simulink model "prey_pred_ext"  (R2023b)
settings: Solver=VariableStepAuto  StartTime=0.0  StopTime=tFinal  RelTol=1e-3
values from neighbouring files (symbols this model uses):
  a1 = 1    [prey_pred_ext_params.m]
  a2 = 1    [prey_pred_ext_params.m]
  b1 = 0.0002    [prey_pred_ext_params.m]
  g1 = 0.01    [prey_pred_ext_params.m]
  g2 = 0.001    [prey_pred_ext_params.m]
  x10 = 3000    [prey_pred_ext_params.m]
  x20 = 1000    [prey_pred_ext_params.m]
settings Model: Creator=martinhaugen  LastModifiedBy=martinhaugen

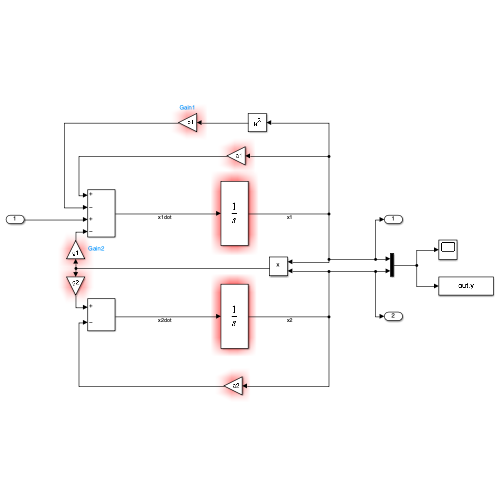
[thumbnail: Simulink's stored preview of the top-level diagram]
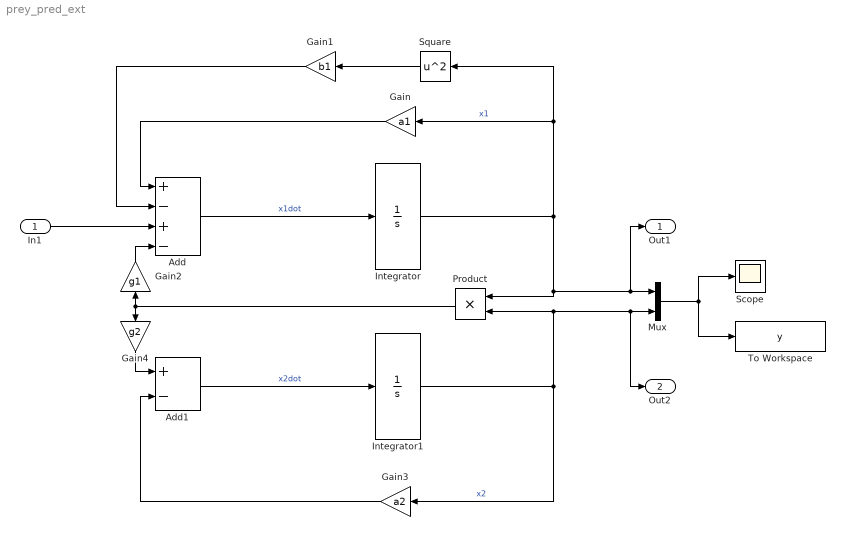
== system prey_pred_ext ==
  In1 : Inport
  Add : Sum  Inputs=+-+-
  Add1 : Sum  Inputs=+-
  Gain : Gain  Gain=a1
  Gain1 : Gain  Gain=b1
  Gain2 : Gain  Gain=g1
  Gain3 : Gain  Gain=a2
  Gain4 : Gain  Gain=g2
  Integrator : Integrator  InitialCondition=x10
  Integrator1 : Integrator  InitialCondition=x20
  Mux : Mux  Inputs=2
  Product : Product
  Scope : Scope
  Square : Math  Operator=square
  To Workspace : ToWorkspace  VariableName=y  SaveFormat=Timeseries  SampleTime=-1
  Out1 : Outport
  Out2 : Outport  Port=2
  wires:
  Add/1 -> Integrator/1  "x1dot"
  Integrator/1 -> Out1/1, Mux/1, Product/1, Square/1, Gain/1  "x1"
  Add1/1 -> Integrator1/1  "x2dot"
  Integrator1/1 -> Gain3/1, Out2/1, Mux/2, Product/2  "x2"
  Gain/1 -> Add/1
  Square/1 -> Gain1/1
  Gain1/1 -> Add/2
  Product/1 -> Gain4/1, Gain2/1
  Gain2/1 -> Add/4
  In1/1 -> Add/3
  Gain3/1 -> Add1/2
  Gain4/1 -> Add1/1
  Mux/1 -> To Workspace/1, Scope/1
